simulink model "Automated_Algorithm"  (R2023a)
settings: Solver=VariableStepAuto  StartTime=0.0  StopTime=10.0  RelTol=1e-3
undefined symbols (not defined in the file): fdesignblkfcn, gcbh
libraries: matrix_library x6, dspstat3 x2, dspsnks4 x1, dspsrcs4 x1
settings Model: Creator=Sam Kramer  LastModifiedBy=Sam Kramer

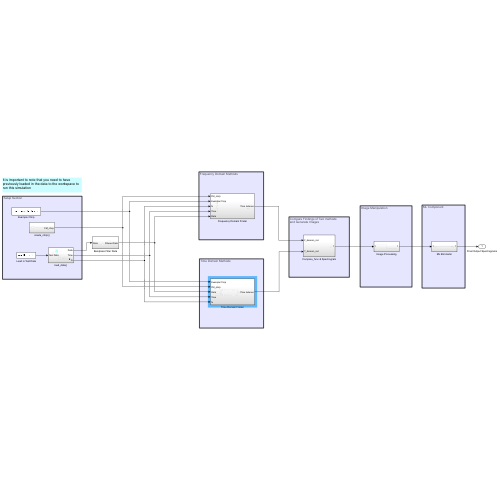
[thumbnail: Simulink's stored preview of the top-level diagram]
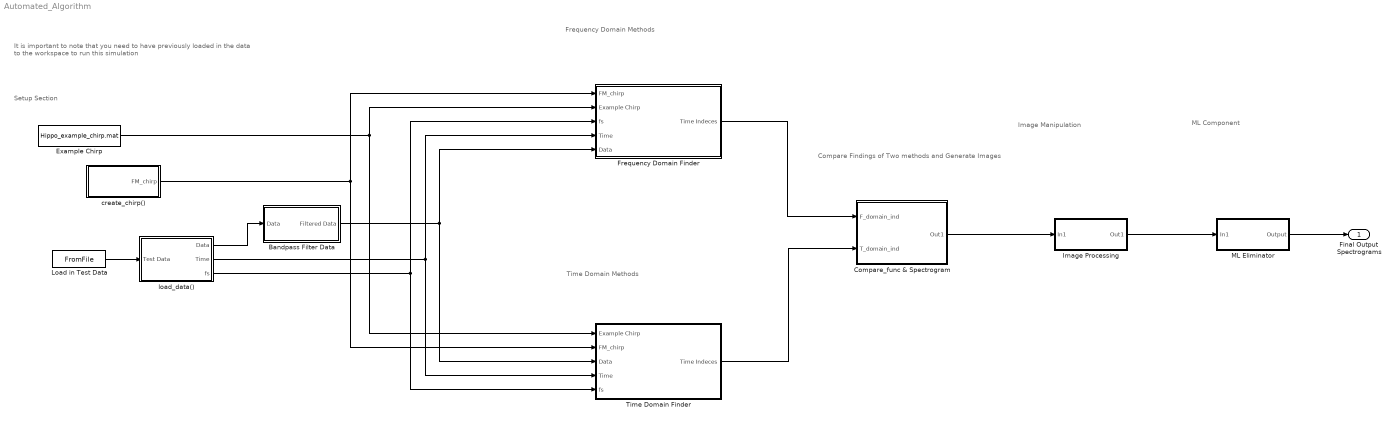
== system Automated_Algorithm ==
  note: It is important to note that you need to have previously loaded in the data to the workspace to run this simulation
  note: Compare Findings of Two methods
      | and Generate Images
  note: ML Component
  note: Image Manipulation
  note: Frequency Domain Methods
  note: Time Domain Methods
  note: Setup Section
  Bandpass Filter Data : Subsystem
  Compare_func & Spectrogram : Subsystem
  Example Chirp : FromFile  FileName=Hippo_example_chirp.mat  SampleTime=0
  Frequency Domain Finder : Subsystem
  Image Processing : Subsystem
  Load in Test Data : FromFile  SampleTime=0
  ML Eliminator : Subsystem
  Time Domain Finder : Subsystem
  create_chirp() : Subsystem
  load_data() : Subsystem
  Final Output Spectrograms : Outport
  wires:
  create_chirp()/1(FM_chirp) -> Frequency Domain Finder/1(FM_chirp), Time Domain Finder/2(FM_chirp)
  load_data()/1(Data) -> Bandpass Filter Data/1(Data)
  load_data()/2(Time) -> Frequency Domain Finder/4(Time), Time Domain Finder/4(Time)
  load_data()/3(fs) -> Frequency Domain Finder/3(fs), Time Domain Finder/5(fs)
  Example Chirp/1 -> Time Domain Finder/1(Example Chirp), Frequency Domain Finder/2(Example Chirp)
  Image Processing/1(Out1) -> ML Eliminator/1(In1)
  Frequency Domain Finder/1(Time Indeces) -> Compare_func & Spectrogram/1(F_domain_ind)
  Time Domain Finder/1(Time Indeces) -> Compare_func & Spectrogram/2(T_domain_ind)
  Compare_func & Spectrogram/1(Out1) -> Image Processing/1(In1)
  ML Eliminator/1(Output) -> Final Output Spectrograms/1
  Load in Test Data/1 -> load_data()/1(Test Data)
  Bandpass Filter Data/1(Filtered Data) -> Time Domain Finder/3(Data), Frequency Domain Finder/5(Data)

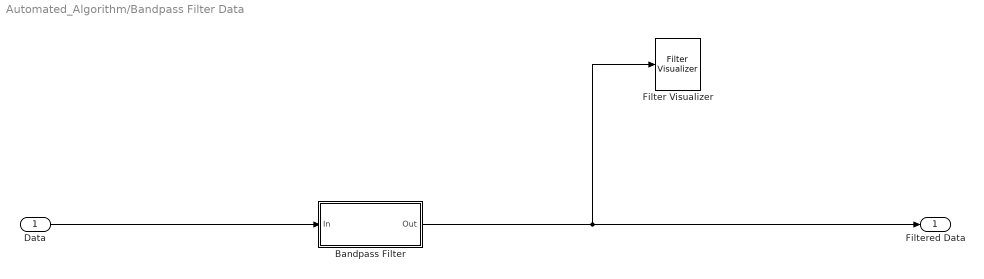
== system Automated_Algorithm/Bandpass Filter Data ==
  Data : Inport
  Bandpass Filter : Subsystem  DialogController=fdesignblkfcn  InitFcn=fdesignblkfcn(gcbh, {'InitFcn'});  mask(Bandpass Filter){}
      mask help: dsp:DSPFilterDesignBlockDialog:BandpassFdesign_MaskDesc
      settings: CopyFcn=fdesignblkfcn(gcbh, {'CopyFcn'});
      mask Help: helpview(mapfilelocation('dsp'), 'dspbandpassfilter');
      mask Display: disp('Bandpass');
  Filter Visualizer : dspsnks4/Filter Visualizer  NumFilters=1  FilterType=FIR  FFTLength=2048  NormalizedFrequency=on  SampleRate=44100  FrequencyRange=[0,1]  XScale=Linear  MagnitudeDisplay=Magnitude (dB)  PlotAsMagnitudePhase=off  PlotType=Line  AxesScaling=Auto  AxesScalingNumUpdates=100  MaximizeAxes=Auto  Title=Magnitude Response  YLimits=[-25,25]  ShowLegend=off  FilterNames=[]  ShowGrid=on  Visible=off  ExpandToolstrip=off
  Filtered Data : Outport
  wires:
  Data/1 -> Bandpass Filter/1(In)
  Bandpass Filter/1(Out) -> Filter Visualizer/1, Filtered Data/1

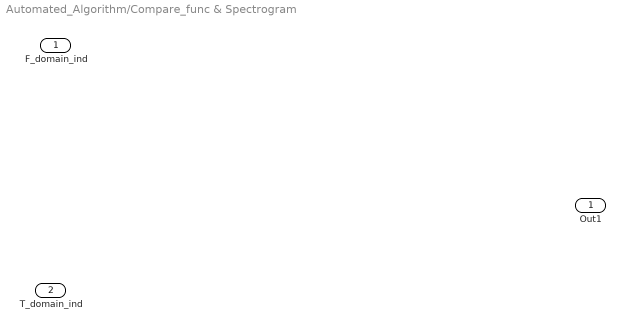
== system Automated_Algorithm/Compare_func & Spectrogram ==
  F_domain_ind : Inport
  T_domain_ind : Inport  Port=2
  Out1 : Outport

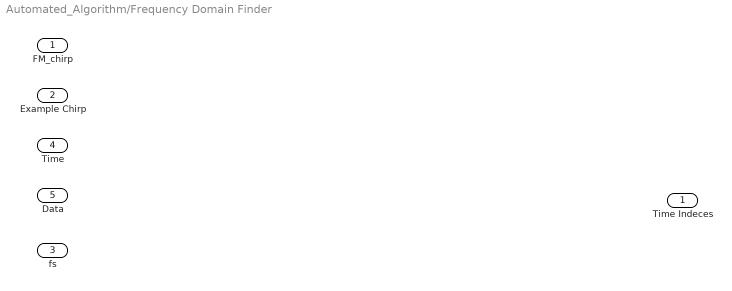
== system Automated_Algorithm/Frequency Domain Finder ==
  FM_chirp : Inport
  Example Chirp : Inport  Port=2
  fs : Inport  Port=3
  Time : Inport  Port=4
  Data : Inport  Port=5
  Time Indeces : Outport

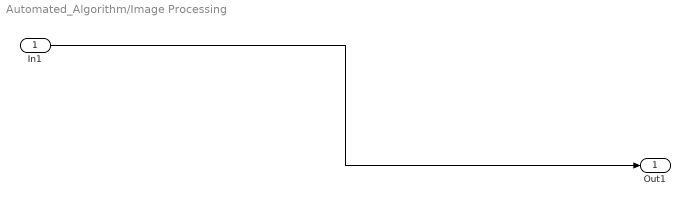
== system Automated_Algorithm/Image Processing ==
  In1 : Inport
  Out1 : Outport
  wires:
  In1/1 -> Out1/1

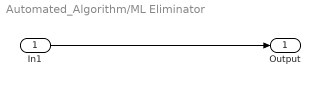
== system Automated_Algorithm/ML Eliminator ==
  In1 : Inport
  Output : Outport
  wires:
  In1/1 -> Output/1

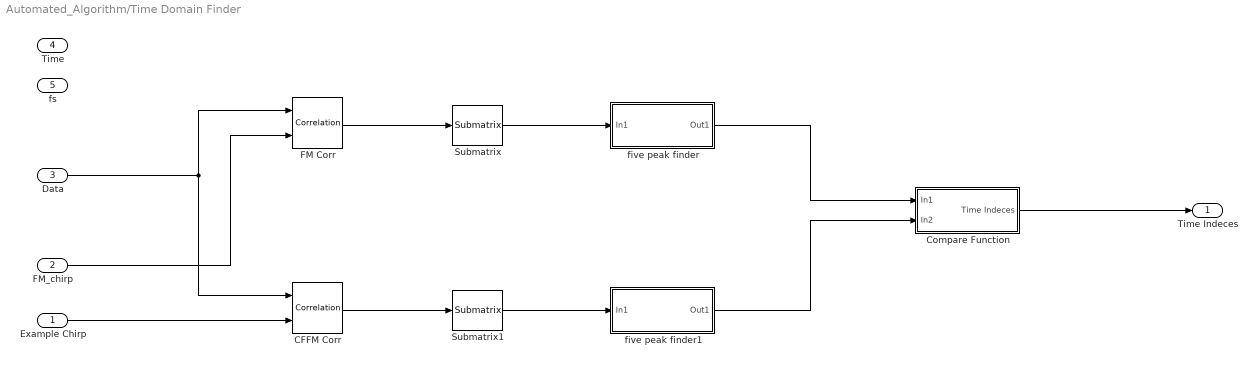
== system Automated_Algorithm/Time Domain Finder ==
  Example Chirp : Inport
  FM_chirp : Inport  Port=2
  Data : Inport  Port=3
  Time : Inport  Port=4
  fs : Inport  Port=5
  CFFM Corr : dspstat3/Correlation  domain=Time  roundingMode=Floor  overflowMode=off  outputDataTypeStr=Inherit: Same as accumulator  outputMin=[]  outputMax=[]  outputLastDataTypeStr=Inherit: Same as accumulator
  Compare Function : Subsystem
  FM Corr : dspstat3/Correlation  domain=Time  roundingMode=Floor  overflowMode=off  outputDataTypeStr=Inherit: Same as accumulator  outputMin=[]  outputMax=[]  outputLastDataTypeStr=Inherit: Same as accumulator
  Submatrix : matrix_library/Submatrix  RowSpan=All rows  RowStartMode=First  RowStartIndex=1  RowEndMode=Last  RowEndIndex=1  ColSpan=Range of columns  ColStartMode=Middle  ColStartIndex=1  ColEndMode=Last  ColEndIndex=1
  Submatrix1 : matrix_library/Submatrix  RowSpan=All rows  RowStartMode=First  RowStartIndex=1  RowEndMode=Last  RowEndIndex=1  ColSpan=Range of columns  ColStartMode=Middle  ColStartIndex=1  ColEndMode=Last  ColEndIndex=1
  five peak finder : Subsystem
  five peak finder1 : Subsystem
  Time Indeces : Outport
  wires:
  FM_chirp/1 -> FM Corr/2
  Data/1 -> CFFM Corr/1, FM Corr/1
  FM Corr/1 -> Submatrix/1
  Example Chirp/1 -> CFFM Corr/2
  CFFM Corr/1 -> Submatrix1/1
  Submatrix/1 -> five peak finder/1(In1)
  Submatrix1/1 -> five peak finder1/1(In1)
  five peak finder/1(Out1) -> Compare Function/1(In1)
  five peak finder1/1(Out1) -> Compare Function/2(In2)
  Compare Function/1(Time Indeces) -> Time Indeces/1

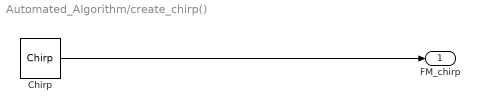
== system Automated_Algorithm/create_chirp() ==
  Chirp : dspsrcs4/Chirp  sweep=Linear  mode=Unidirectional  f0=120000  f1=100000  t1=1  Tsweep=1  phase=0  Ts=1/500000  spf=500000*0.005  datatype=Double  OutputFrames=off
  FM_chirp : Outport
  wires:
  Chirp/1 -> FM_chirp/1

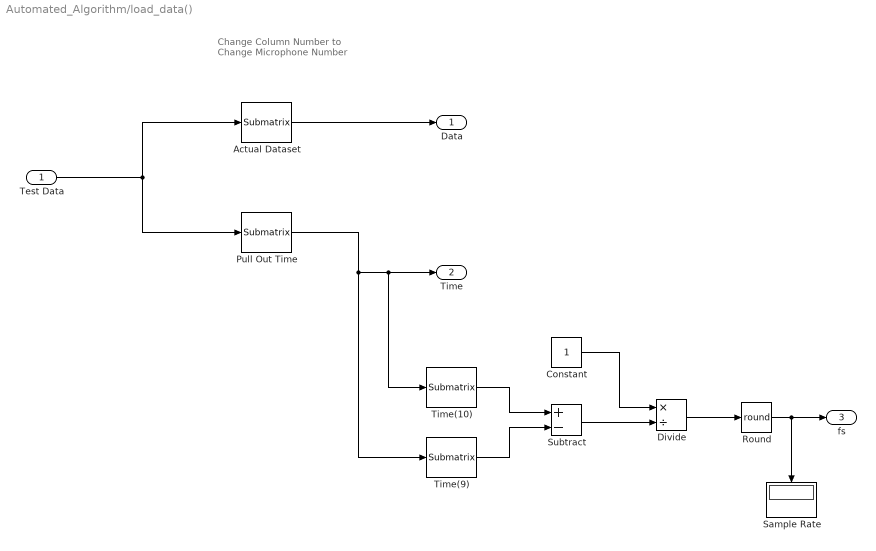
== system Automated_Algorithm/load_data() ==
  note: Change Column Number
      | to Change Microphone Number
  Test Data : Inport
  Actual Dataset : matrix_library/Submatrix  RowSpan=All rows  RowStartMode=First  RowStartIndex=1  RowEndMode=Last  RowEndIndex=1  ColSpan=One column  ColStartMode=Index  ColStartIndex=2  ColEndMode=Last  ColEndIndex=1
  Constant : Constant
  Divide : Product  Inputs=*/
  Pull Out Time : matrix_library/Submatrix  RowSpan=All rows  RowStartMode=First  RowStartIndex=1  RowEndMode=Last  RowEndIndex=1  ColSpan=All columns  ColStartMode=First  ColStartIndex=1  ColEndMode=Last  ColEndIndex=1
  Round : Rounding  Operator=round
  Sample Rate : Display
  Subtract : Sum  Inputs=+-
  Time(10) : matrix_library/Submatrix  RowSpan=One row  RowStartMode=Index  RowStartIndex=10  RowEndMode=Last  RowEndIndex=1  ColSpan=All columns  ColStartMode=First  ColStartIndex=1  ColEndMode=Last  ColEndIndex=1
  Time(9) : matrix_library/Submatrix  RowSpan=One row  RowStartMode=Index  RowStartIndex=9  RowEndMode=Last  RowEndIndex=1  ColSpan=All columns  ColStartMode=First  ColStartIndex=1  ColEndMode=Last  ColEndIndex=1
  Data : Outport
  Time : Outport  Port=2
  fs : Outport  Port=3
  wires:
  Test Data/1 -> Pull Out Time/1, Actual Dataset/1
  Actual Dataset/1 -> Data/1
  Pull Out Time/1 -> Time(10)/1, Time/1, Time(9)/1
  Time(9)/1 -> Subtract/2
  Time(10)/1 -> Subtract/1
  Constant/1 -> Divide/1
  Subtract/1 -> Divide/2
  Divide/1 -> Round/1
  Round/1 -> fs/1, Sample Rate/1

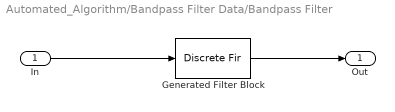
== system Automated_Algorithm/Bandpass Filter Data/Bandpass Filter ==
  In : Inport
  Generated Filter Block : DiscreteFir  Tag=BlockMethodSubSystem  Coefficients=[-0.00089922914877444424 0.00164145187479435928 0.00313520718422255745 -0.00407075508288146874 -0.00637318522279040241 0.00748742868060905172 0.00983543195662957281 -0.0101893165134462078 -0.011302794465874122 0.0096929185841818314 0.00794286539874642684 -0.00313682478812214987 0.00282998788779430157 -0.0115086742430014887 -0.0220801362194615741 0.0342453254245076721 0.0483566616489054524 -0.0623553691698842255 -0.0775034781625938557 0.0906877681531256252 0.103531711058441514 -0.112978600842298299 -0.120358660249784491 0.123793608015391313 0.123793608015391313 -0.120358660249784491 -0.112978600842298299 0.103531711058441514 0.0906877681531256252 -0.0775034781625938557 -0.0623553691698842255 0.0483566616489054524 0.0342453254245076721 -0.0220801362194615741 -0.0115086742430014887 0.00282998788779430157 -0.00313682478812214987 0.00794286539874642684 0.0096929185841818314 -0.011302794465874122 -0.0101893165134462078 0.00983543195662957281 0.00748742868060905172 -0.00637318522279040241 -0.00407075508288146874 0.00313520718422255745 0.00164145187479435928 -0.00089922914877444424]  InputProcessing=Columns as channels (frame based)
  Out : Outport  VectorParamsAs1DForOutWhenUnconnected=off
  wires:
  In/1 -> Generated Filter Block/1
  Generated Filter Block/1 -> Out/1

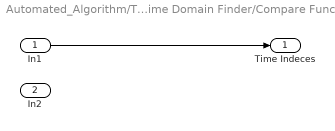
== system Automated_Algorithm/Time Domain Finder/Compare Function ==
  In1 : Inport
  In2 : Inport  Port=2
  Time Indeces : Outport
  wires:
  In1/1 -> Time Indeces/1

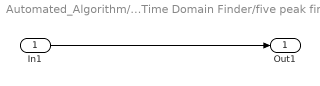
== system Automated_Algorithm/Time Domain Finder/five peak finder ==
  In1 : Inport
  Out1 : Outport
  wires:
  In1/1 -> Out1/1

== system Automated_Algorithm/Time Domain Finder/five peak finder1 ==
  In1 : Inport
  Out1 : Outport
  wires:
  In1/1 -> Out1/1
